simulink model "JointSpaceInverseDynamics"  (R2022b)
settings: Solver=VariableStepAuto  StartTime=0.0  StopTime=10.0  RelTol=1e-3
values from neighbouring files (symbols this model uses):
  Kd = [[30,0,0] ... (first row only)    [parameters.m]
  Kp = [[200,0,0] ... (first row only)    [parameters.m]
libraries: robotcorelib x1
settings Model: Creator=uzair  LastModifiedBy=uzair

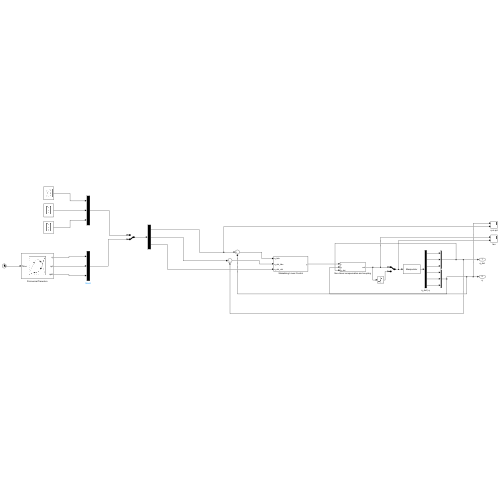
[thumbnail: Simulink's stored preview of the top-level diagram]
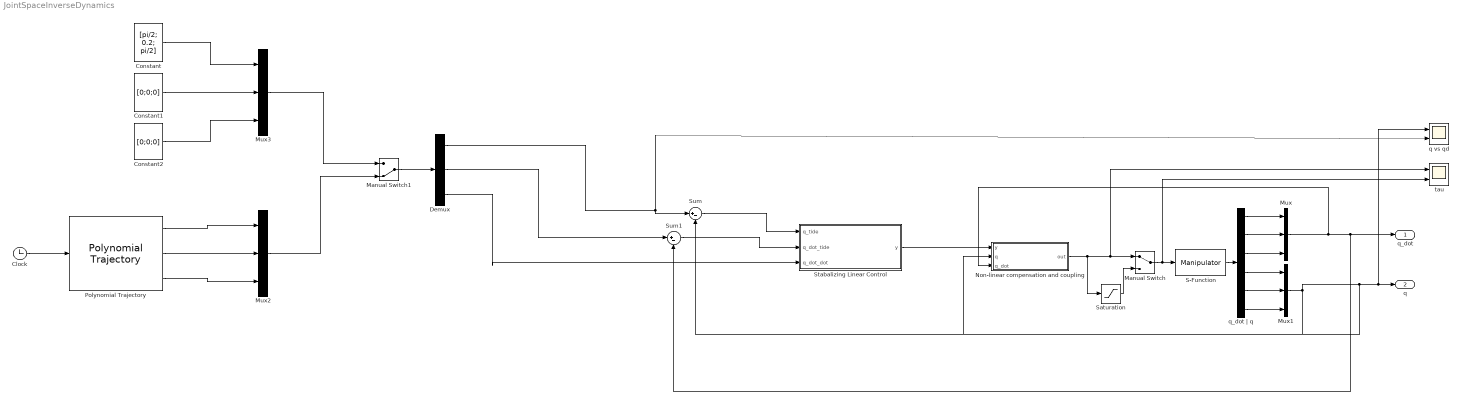
== system JointSpaceInverseDynamics ==
  Clock : Clock
  Constant : Constant  Value=[pi/2; 0.2; pi/2]  VectorParams1D=off
  Constant1 : Constant  Value=[0;0;0]  VectorParams1D=off
  Constant2 : Constant  Value=[0;0;0]  VectorParams1D=off
  Demux : Demux  Outputs=3
  Manual Switch : ManualSwitch
  Manual Switch1 : ManualSwitch  CurrentSetting=0
  Mux{,1..3} (4 alike) : Mux  Inputs=3
  Non-linear compensation and coupling : Subsystem
  Polynomial Trajectory : robotcorelib/Polynomial Trajectory  WaypointSource=Internal  Waypoints=[pi/2,-pi/2,pi/2; -0.2,0.2,-0.2; -pi/2,pi/2,-pi/2]  TimePoints=[ 1, 6, 9 ]  TimeInterval=[ 1, 4 ]  Method=Quintic Polynomial  ParameterSource=Internal  VelocityBoundaryCondition=zeros( 3,3 )  AccelerationBoundaryCondition=zeros( 3,3 )  SimulateUsing=Interpreted execution
  S-Function : S-Function  FunctionName=Manipulator  Parameters=params  SFunctionDeploymentMode=off  EnableBusSupport=off
  Saturation : Saturate  UpperLimit=10  LowerLimit=-10
  Stabalizing Linear Control : Subsystem
  Sum : Sum  Inputs=|+-
  Sum1 : Sum  Inputs=|+-
  q vs qd : Scope  NumInputPorts=2
  q_dot | q : Demux  Outputs=6
  tau : Scope  NumInputPorts=2
  q_dot : Outport
  q : Outport  Port=2
  wires:
  Stabalizing Linear Control/1(y) -> Non-linear compensation and coupling/1(y)
  S-Function/1 -> q_dot | q/1
  q_dot | q/1 -> Mux/1
  q_dot | q/2 -> Mux/2
  q_dot | q/3 -> Mux/3
  q_dot | q/6 -> Mux1/3
  q_dot | q/5 -> Mux1/2
  q_dot | q/4 -> Mux1/1
  Mux/1 -> Non-linear compensation and coupling/3(q_dot), q_dot/1, Sum1/2
  Mux1/1 -> Non-linear compensation and coupling/2(q), q vs qd/1, q/1, Sum/2
  Sum/1 -> Stabalizing Linear Control/1(q_tide)
  Sum1/1 -> Stabalizing Linear Control/2(q_dot_tide)
  Clock/1 -> Polynomial Trajectory/1
  Manual Switch/1 -> tau/2, S-Function/1
  Non-linear compensation and coupling/1(out) -> Saturation/1, tau/1, Manual Switch/1
  Saturation/1 -> Manual Switch/2
  Polynomial Trajectory/1 -> Mux2/1
  Polynomial Trajectory/2 -> Mux2/2
  Polynomial Trajectory/3 -> Mux2/3
  Constant/1 -> Mux3/1
  Constant1/1 -> Mux3/2
  Constant2/1 -> Mux3/3
  Mux3/1 -> Manual Switch1/1
  Mux2/1 -> Manual Switch1/2
  Manual Switch1/1 -> Demux/1
  Demux/1 -> q vs qd/2, Sum/1
  Demux/2 -> Sum1/1
  Demux/3 -> Stabalizing Linear Control/3(q_dot_dot)

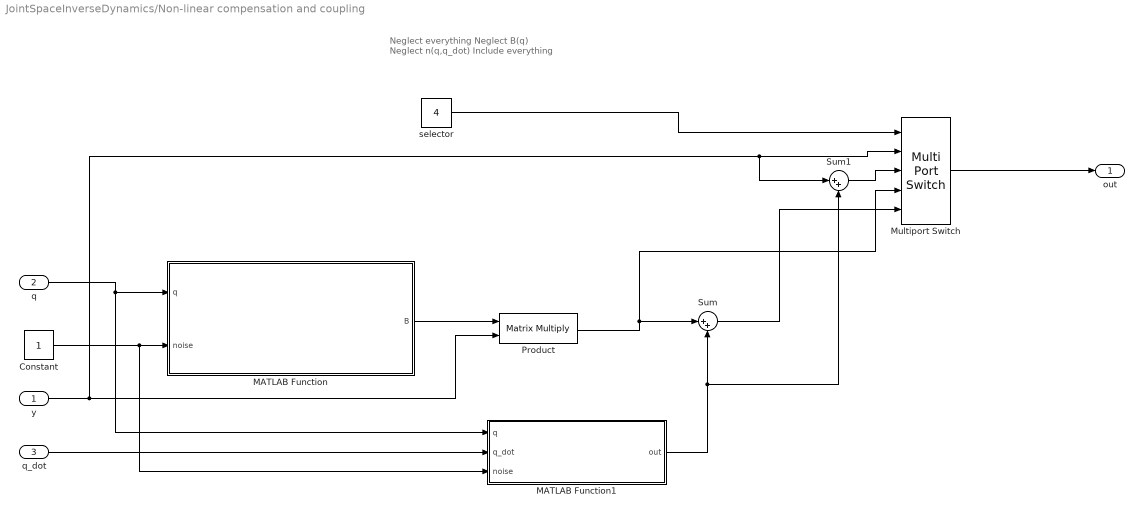
== system JointSpaceInverseDynamics/Non-linear compensation and coupling ==
  note: Neglect everything
      | Neglect B(q)
      | Neglect n(q,q_dot)
      | Include everything
  y : Inport
  q : Inport  Port=2
  q_dot : Inport  Port=3
  Constant : Constant
  MATLAB Function : MATLAB Function  TreatAsAtomicUnit=on
  MATLAB Function1 : MATLAB Function  TreatAsAtomicUnit=on
  Multiport Switch : MultiPortSwitch  Inputs=4  SaturateOnIntegerOverflow=off  InputSameDT=off
  Product : Product  Multiplication=Matrix(*)
  Sum : Sum  Inputs=|++
  Sum1 : Sum  Inputs=|++
  selector : Constant  Value=4
  out : Outport
  wires:
  q/1 -> MATLAB Function1/1(q), MATLAB Function/1(q)
  MATLAB Function/1(B) -> Product/1
  y/1 -> Sum1/1, Multiport Switch/2, Product/2
  Product/1 -> Multiport Switch/4, Sum/1
  q_dot/1 -> MATLAB Function1/2(q_dot)
  MATLAB Function1/1(out) -> Sum1/2, Sum/2
  Constant/1 -> MATLAB Function1/3(noise), MATLAB Function/2(noise)
  selector/1 -> Multiport Switch/1
  Multiport Switch/1 -> out/1
  Sum1/1 -> Multiport Switch/3
  Sum/1 -> Multiport Switch/5

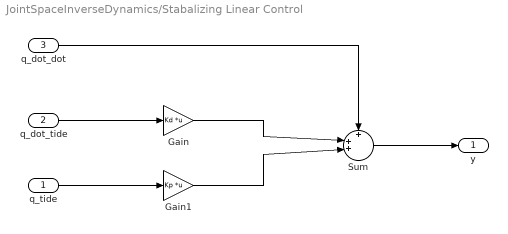
== system JointSpaceInverseDynamics/Stabalizing Linear Control ==
  q_tide : Inport
  q_dot_tide : Inport  Port=2
  q_dot_dot : Inport  Port=3
  Gain : Gain  Gain=Kd  Multiplication=Matrix(K*u)
  Gain1 : Gain  Gain=Kp  Multiplication=Matrix(K*u)
  Sum : Sum  Inputs=+|++||
  y : Outport
  wires:
  q_tide/1 -> Gain1/1
  q_dot_dot/1 -> Sum/1
  Gain1/1 -> Sum/3
  Sum/1 -> y/1
  q_dot_tide/1 -> Gain/1
  Gain/1 -> Sum/2

== matlab function JointSpaceInverseDynamics/Non-linear compensation and coupling/MATLAB Function1 ==
  data: q input; out output; q_dot input; params parameter; noise input
function out = n(q, q_dot, params, noise)
    
    m1 = params.m(1) * noise;
    m2 = params.m(2) * noise;
    m3 = params.m(3) * noise;

    q1 = q(1);
    q2 = q(2);
    q3 = q(3);

    q1_dot = q_dot(1);
    q2_dot = q_dot(2);
    q3_dot = q_dot(3);

    g = params.g;

    Fv = params.Fv;
 
    B = [[(195791581307*m1)/1220703125000 + (8503*m2)/40000 + (321279862557*m3)/1220703125000 + (8*m3*cos(q3)^2)/625 + (3*m2*q2)/10 + (3*m3*q2)/5 + m2*q2^2 + m3*q2^2 + (8*m3*cos(q3))/125, (2*m2)/5 + (2*m3)/5 + (2*m3*cos(q3))/25, (2*m3*sin(q3)*(q2 + 3/10))/25]
        [                                                                                                                                         (2*m2)/5 + (2*m3)/5 + (2*m3*cos(q3))/25,                                 m2 + m3,                             0]
        [                                                                                                                                                   (2*m3*sin(q3)*(q2 + 3/10))/25,                                       0,            (32637*m3)/1562500]];

    C = [[q2_dot*((3*m2)/20 + (3*m3)/10 + m2*q2 + m3*q2) - q3_dot*((4*m3*sin(2*q3))/625 + (4*m3*sin(q3))/125), q1_dot*((3*m2)/20 + (3*m3)/10 + m2*q2 + m3*q2), (2*m3*q3_dot*cos(q3)*(q2 + 3/10))/25 - q1_dot*((4*m3*sin(q3))/125 + (8*m3*cos(q3)*sin(q3))/625)]
        [                        -q1_dot*((3*m2)/20 + (3*m3)/10 + m2*q2 + m3*q2) - (2*m3*q3_dot*sin(q3))/25,                                              0,                                                                       -(2*m3*q1_dot*sin(q3))/25]
        [                      q1_dot*((4*m3*sin(2*q3))/625 + (4*m3*sin(q3))/125) + (2*m3*q2_dot*sin(q3))/25,                       (2*m3*q1_dot*sin(q3))/25,                                                                                               0]];

    G = [(g*m1*cos(q1))/5 - g*m2*((3*sin(q1))/20 - (2*cos(q1))/5 + q2*sin(q1)) + g*m3*((2*cos(q1))/5 + (2*cos(q1)*cos(q3))/25 - sin(q1)*(q2 + 3/10));
                                                                                                                        g*cos(q1)*(m2 + m3);
                                                                                                               -(2*g*m3*sin(q1)*sin(q3))/25];

    out = C*q_dot + diag(Fv)*q_dot + G;
end

== matlab function JointSpaceInverseDynamics/Non-linear compensation and coupling/MATLAB Function ==
  data: q input; B output; params parameter; noise input
function B = inertiaMatrix(q, params, noise)
    q1 = q(1); % not used in this matrix
    q2 = q(2);
    q3 = q(3);

    m1 = params.m(1) * noise;
    m2 = params.m(2) * noise;
    m3 = params.m(3) * noise;

    B = [[(195791581307*m1)/1220703125000 + (8503*m2)/40000 + (321279862557*m3)/1220703125000 + (8*m3*cos(q3)^2)/625 + (3*m2*q2)/10 + (3*m3*q2)/5 + m2*q2^2 + m3*q2^2 + (8*m3*cos(q3))/125, (2*m2)/5 + (2*m3)/5 + (2*m3*cos(q3))/25, (2*m3*sin(q3)*(q2 + 3/10))/25]
        [                                                                                                                                         (2*m2)/5 + (2*m3)/5 + (2*m3*cos(q3))/25,                                 m2 + m3,                             0]
        [                                                                                                                                                   (2*m3*sin(q3)*(q2 + 3/10))/25,                                       0,            (32637*m3)/1562500]];
end
